simulink model "velocity_control"  (R2019a)
settings: Solver=ode1  StartTime=0.0  StopTime=Inf  FixedStep=0.001  RelTol=1e-3
PostLoadFcn:
  | , if any(exist('dsrtsu_mdlpostloadfcn', 'file') == [2, 3, 6]), try dsrtsu_mdlpostloadfcn('Execute', bdroot); catch fprintf('Error in PostLoadFcn (dsrtsu_mdlpostloadfcn) for model "%s":\n %s\n', bdroot, lasterr); end, end,
settings Model: DSRTSU_INTERNAL_RTI_VER=480  DSRTSU_INTERNAL_RTI_TYPE=rti1401  Creator=zhou  LastModifiedBy=86185
settings DataIOCC: ReturnWorkspaceOutputs=off
settings OptimizationCC: BlockReduction=off  OptimizeBlockIOStorage=off  BufferReuse=off  GlobalBufferReuse=off  ExpressionFolding=off  LocalBlockOutputs=off  OptimizeDataStoreBuffers=off  BusAssignmentInplaceUpdate=off
settings DebuggingCC: ArithmeticOperatorsInVariantConditions=warning
settings HardwareCC: ProdBitPerPointer=32  ProdBitPerSizeT=32  ProdBitPerPtrDiffT=32  ProdLargestAtomicInteger=Integer  ProdEndianess=BigEndian  ProdWordSize=32  ProdHWDeviceType=Custom Processor->Custom  TargetIntDivRoundTo=Zero  TargetEndianess=BigEndian  TargetHWDeviceType=Custom Processor->Custom
settings SFSimCC: SimUseLocalCustomCode=off
settings RTWCC: SystemTargetFile=rti1401.tlc  MakeCommand=make_rti  TemplateMakefile=rti1401.tmf  Description=dSPACE DS1401 Hardware Platform  RTWUseLocalCustomCode=off
settings CodeAppCC: StateflowObjectComments=on
settings STFCustomTargetCC: ParMdlRefBuildCompliant=on  MatFileLogging=on  GRTInterface=off  SystemTargetFile=rti1401.tlc
settings GRTTargetCC: TargetLangStandard=C89/C90 (ANSI)  CompOptLevelCompliant=off  ConcurrentExecutionCompliant=off  CombineOutputUpdateFcns=off  CPPClassGenCompliant=off  UseToolchainInfoCompliant=off
settings ConfigComp: CovMetricSettings=dswe

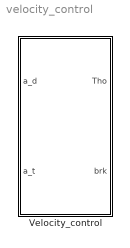
== system velocity_control ==
  Velocity_control : Subsystem

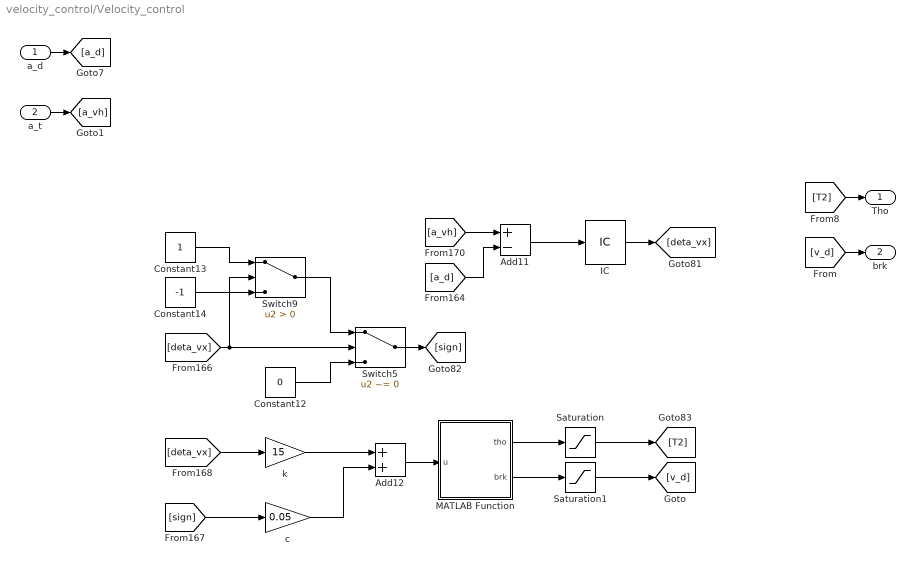
== system velocity_control/Velocity_control ==
  a_d : Inport
  a_t : Inport  Port=2
  Add11 : Sum  Inputs=+-
  Add12 : Sum
  Constant12 : Constant  Value=0
  Constant13 : Constant
  Constant14 : Constant  Value=-1
  IC : InitialCondition  Value=0
  MATLAB Function : MATLAB Function  TreatAsAtomicUnit=on
  Saturation : Saturate  UpperLimit=1  LowerLimit=0
  Saturation1 : Saturate  UpperLimit=0  LowerLimit=-8
  Switch5 : Switch  Criteria=u2 ~= 0
  Switch9 : Switch  Criteria=u2 > Threshold
  c : Gain  Gain=0.05
  k : Gain  Gain=15
  Tho : Outport
  brk : Outport  Port=2
  wires:
  MATLAB Function/1(tho) -> Saturation/1
  a_d/1 -> [a_d]
  [T2] -> Tho/1
  a_t/1 -> [a_vh]
  Constant13/1 -> Switch9/1
  [a_d] -> Add11/2
  Add11/1 -> IC/1
  [deta_vx] -> k/1
  Switch5/1 -> [sign]
  [sign] -> c/1
  Constant14/1 -> Switch9/3
  k/1 -> Add12/1
  c/1 -> Add12/2
  [deta_vx] -> Switch9/2, Switch5/2
  [a_vh] -> Add11/1
  IC/1 -> [deta_vx]
  Switch9/1 -> Switch5/1
  Constant12/1 -> Switch5/3
  [v_d] -> brk/1
  Add12/1 -> MATLAB Function/1(u)
  MATLAB Function/2(brk) -> Saturation1/1
  Saturation/1 -> [T2]
  Saturation1/1 -> [v_d]

== matlab function velocity_control/Velocity_control/MATLAB Function ==
  data: u input; tho output; brk output
function [tho,brk] = fcn(u)
if u >= 0
    brk = 0;
    tho=0.01*u;
else
    tho=0;
    brk = 0.4*u;
end
